simulink model "RL_controller_"  (R2022b)
settings: Solver=VariableStepAuto  StartTime=0.0  StopTime=inf  FixedStep=0.001  MaxStep=0.001  RelTol=1e-3
InitFcn:
  | ro = 0.1 ;
  | 
  | Ku = 9;
  | Tu = 4;
  | Kpmin = 0.32*Ku;
  | Kpmax = 0.6*Ku;
  | Kdmin = 0.08*Ku*Tu;
  | Kdmax = 0.15*Ku*Tu;
libraries: slpidlib x1, rllib x1, simulink x1
settings Model: SimulationMode=accelerator  Creator=Notebook  LastModifiedBy=Administrator
settings SolverCC: AlgebraicLoopSolver=TrustRegion
settings DebuggingCC: ArithmeticOperatorsInVariantConditions=warning
settings ModelReferenceCC: EnableRefExpFcnMdlSchedulingChecks=on
settings SFSimCC: CustomCodeUndefinedFunction=UseInterfaceOnly

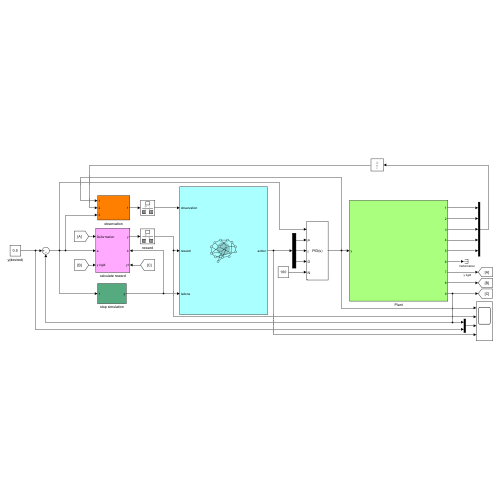
[thumbnail: Simulink's stored preview of the top-level diagram]
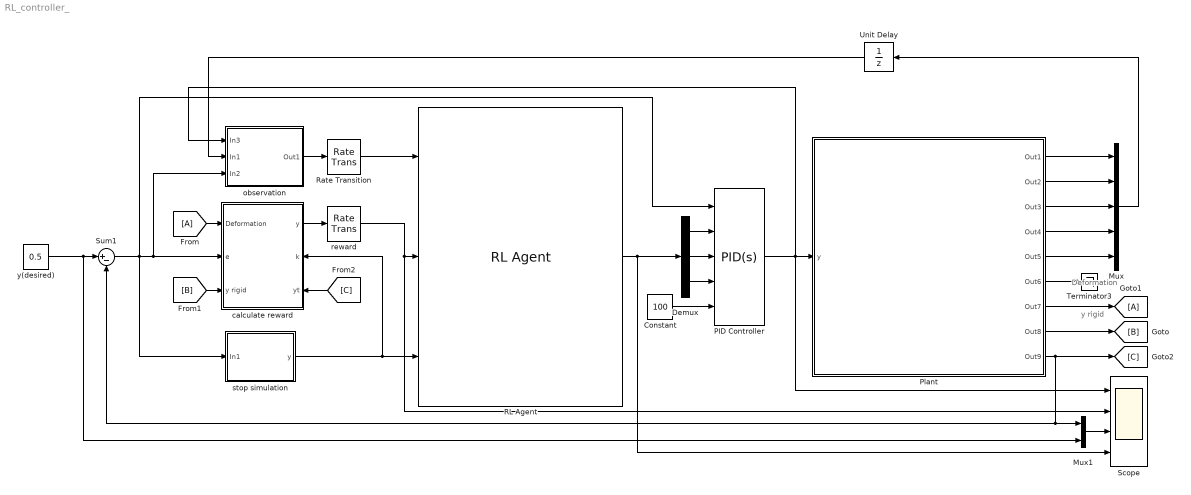
== system RL_controller_ ==
  note: Deformation
  note: y rigid
  Constant : Constant  Value=100
  Demux : Demux  Outputs=3
  From : From
  Goto1 : Goto
  Mux : Mux  Inputs=5
  Mux1 : Mux  Inputs=2
  PID Controller : slpidlib/PID Controller  Controller=PID  Form=Parallel  TimeDomain=Continuous-time  UseExternalTs=off  SampleTime=-1  IntegratorMethod=Forward Euler  FilterMethod=Forward Euler  ControllerParametersSource=external  P=1  I=1  UseKiTs=off  D=0  N=100  UseFilter=on  TunerSelectOption=Transfer Function Based (PID Tuner App)  InitialConditionSource=internal  InitialConditionForIntegrator=0  InitialConditionForFilter=0  DifferentiatorICPrevScaledInput=0  ExternalReset=none  TrackingMode=off  Kt=1  LimitOutput=off  SatLimitsSource=internal  UpperSaturationLimit=inf  LowerSaturationLimit=-inf  LinearizeAsGain=on  AntiWindupMode=none  Kb=1  LimitIntegrator=off  UpperIntegratorSaturationLimit=inf  LowerIntegratorSaturationLimit=-inf  POutMin=[]  POutMax=[]  IOutMin=[]  IOutMax=[]  DOutMin=[]  DOutMax=[]  NOutMin=[]  NOutMax=[]  SumOutMin=[]  SumOutMax=[]  SaturationOutMin=[]  SaturationOutMax=[]  PParamMin=[]  PParamMax=[]  IParamMin=[]  IParamMax=[]  DParamMin=[]  DParamMax=[]  NParamMin=[]  NParamMax=[]  KbParamMin=[]  KbParamMax=[]  KtParamMin=[]  KtParamMax=[]  KbOutMin=[]  KbOutMax=[]  KtOutMin=[]  KtOutMax=[]  IntegratorOutMin=[]  IntegratorOutMax=[]  FilterOutMin=[]  FilterOutMax=[]  SumI1OutMin=[]  SumI1OutMax=[]  SumI2OutMin=[]  SumI2OutMax=[]  SumI3OutMin=[]  SumI3OutMax=[]  SumI4OutMin=[]  SumI4OutMax=[]  SumDOutMin=[]  SumDOutMax=[]  DifferentiatorOutMin=[]  DifferentiatorOutMax=[]  FilterDiffOutCoefMin=[]  FilterDiffOutCoefMax=[]  ReciprocalOutMin=[]  ReciprocalOutMax=[]  SumDenOutMin=[]  SumDenOutMax=[]  SumNumOutMin=[]  SumNumOutMax=[]  DivideOutMin=[]  DivideOutMax=[]  UdiffTsProdOutMin=[]  UdiffTsProdOutMax=[]  NTsProdOutMin=[]  NTsProdOutMax=[]  UintegralTsProdOutMin=[]  UintegralTsProdOutMax=[]  UngainTsProdOutMin=[]  UngainTsProdOutMax=[]  ClampingZeroOutDataTypeStr=Inherit: Inherit via back propagation  ClampingZeroOutMin=[]  ClampingZeroOutMax=[]  FilterDenConstantOutDataTypeStr=Inherit: Inherit via back propagation  FilterDenConstantOutMin=[]  FilterDenConstantOutMax=[]  PCopyOutDataTypeStr=Inherit: Inherit via back propagation  PCopyOutMin=[]  PCopyOutMax=[]  NCopyOutDataTypeStr=Inherit: Inherit via back propagation  NCopyOutMin=[]  NCopyOutMax=[]  IntegratorContinuousStateAttributes=''  IntegratorStateMustResolveToSignalObject=off  IntegratorRTWStateStorageClass=Auto  FilterContinuousStateAttributes=''  FilterStateMustResolveToSignalObject=off  FilterRTWStateStorageClass=Auto  ParallelPVariant=ExternalParameters  IdealPVariant=Disabled  IVariant=ExternalParameters  DVariant=ExternalParameters  IntegratorVariant=Continuous  SatVariant=Disabled  AWVariant=Passthrough  PCopyVariant=Disabled  TRVariant=Disabled  FdbkBlocksVariant=Forward  IdealPFdbkVariant=Disabled  SatFdbkVariant=Disabled  DerivativeFilterVariant=ContFilter  NVariant=ExternalParameters  NCopyVariant=Disabled  FilterICVariant=InternalICsFilter  IntegratorICVariant=InternalICs  ExternalResetVariant=Disabled  TRSumVariant=Passthrough  SumFdbkVariant=Disabled  SumVariant=Sum_PID  TsampFilterVariant=InternalTs  TsampNgainVariant=Passthrough  TsampIntegralVariant=Passthrough  ExternalSaturationOutDataTypeStr=Inherit: Same as second input
  Plant : Subsystem
  RL Agent : rllib/RL Agent  Agent=agent  ExternalActionAsInput=off  ProvideLastAction=off  ProvideCumRwd=off  TreatAsDirectFeedthrough=on  UseStrictObservationDataTypes=off
  Rate Transition : RateTransition
  Scope : Scope  NumInputPorts=4
  Sum1 : Sum  Inputs=|+-
  Terminator3 : Terminator
  Unit Delay : UnitDelay  SampleTime=-1  HasFrameUpgradeWarning=on
  calculate reward : Subsystem
      settings: PortSchema="{\"entries\":[{\"content\":{\"sides\":[{\"content\":{\"connectorIds\":[\"In1\",\"In2\",\"In3\"]},\"type\":\"ConnectorPlacement.EquallySpacedRectSide\",\"uuid\":\"6d7fc479-8b54-4eda-9f6d-c70e7c76a1e2\"},{\"content\":{\"connectorIds\":[\"Out1\",\"In4\",\"In5\"],\"side\":\"RIGHT\"},\"type\":\"ConnectorPlacement.EquallySpacedRectSide\",\"uuid\":\"b691a02b-c792-4e07-977e-e9bf68ac6416\"},{\"content\":{\"connectorIds\":[],\"side\":\"TOP\"},\"type\":\"ConnectorPlacement.EquallySpacedRectSide\",\"uuid\":\"d0b1642a-ff91-438e-8bf3-0ab91db4c543\"}]},\"type\":\"ConnectorPlacement.EquallySpacedConnector\",\"uuid\":\"cdcc6e51-e785-4fe5-9481-e2f237055900\"}],\"packageUris\":[\"http://schema.mathworks.com/mf0/Connector/R2020b\"],\"version\":\"1.0\"}"
  observation : Subsystem
  reward : RateTransition
  stop simulation : Subsystem
  y(desired) : Constant  Value=0.5
  wires:
  Sum1/1 -> observation/3(In2), calculate reward/2(e), stop simulation/1(In1), PID Controller/1
  y(desired)/1 -> Mux1/2, Sum1/1
  calculate reward/1(y) -> reward/1
  observation/1(Out1) -> Rate Transition/1
  Rate Transition/1 -> RL Agent/1
  reward/1 -> RL Agent/2, Scope/2
  stop simulation/1(y) -> RL Agent/3, calculate reward/4(k)
  Plant/1(Out1) -> Mux/1
  Plant/2(Out2) -> Mux/2
  Plant/9(Out9) -> [C], Mux1/1, Sum1/2
  Plant/7(Out7) -> Goto1/1
  Plant/8(Out8) -> [B]
  From/1 -> calculate reward/1(Deformation)
  [B] -> calculate reward/3(y rigid)
  Mux/1 -> Unit Delay/1
  Mux1/1 -> Scope/3
  Plant/3(Out3) -> Mux/3
  [C] -> calculate reward/5(yt)
  Unit Delay/1 -> observation/2(In1)
  Plant/5(Out5) -> Mux/5
  Plant/6(Out6) -> Terminator3/1
  Plant/4(Out4) -> Mux/4
  PID Controller/1 -> observation/1(In3), Plant/1(y), Scope/1
  Demux/1 -> PID Controller/2
  Demux/2 -> PID Controller/3
  Demux/3 -> PID Controller/4
  RL Agent/1 -> Demux/1, Scope/4
  Constant/1 -> PID Controller/5

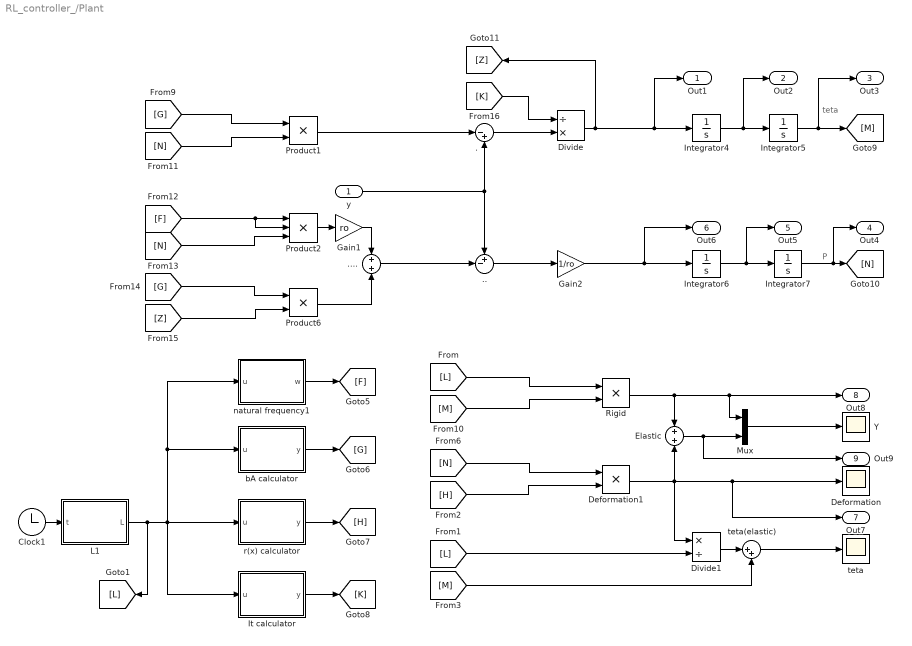
== system RL_controller_/Plant ==
  note: P
  note: teta
  y : Inport
  . : Sum  Inputs=|-+
  .. : Sum  Inputs=+-|
  .... : Sum  Inputs=+|+
  Clock1 : Clock
      settings: Decimation=2
  Deformation : Scope
  Deformation1 : Product
  Divide : Product  Inputs=/*
  Divide1 : Product  Inputs=*/
  Elastic : Sum  Inputs=+|+
  Gain1 : Gain  Gain=ro
  Gain2 : Gain  Gain=1/ro
  Integrator{4..7} (4 alike) : Integrator
  It calculator : MATLAB Function  TreatAsAtomicUnit=on
  L1 : MATLAB Function  TreatAsAtomicUnit=on
  Mux : Mux  Inputs=2
  Product1 : Product
  Product2 : Product  Inputs=3
  Product6 : Product
  Rigid : Product
  Y : Scope
  bA calculator : MATLAB Function  TreatAsAtomicUnit=on
  natural frequency1 : MATLAB Function  TreatAsAtomicUnit=on
  r(x) calculator : MATLAB Function  TreatAsAtomicUnit=on
  teta : Scope
  teta(elastic) : Sum  Inputs=|++
  Out1 : Outport
  Out2 : Outport  Port=2
  Out3 : Outport  Port=3
  Out4 : Outport  Port=4
  Out5 : Outport  Port=5
  Out6 : Outport  Port=6
  Out7 : Outport  Port=7
  Out8 : Outport  Port=8
  Out9 : Outport  Port=9
  wires:
  teta(elastic)/1 -> teta/1
  Integrator6/1 -> Out5/1, Integrator7/1
  [N] -> Product1/2
  [L] -> Rigid/1
  ./1 -> Divide/2
  [Z] -> Product6/2
  bA calculator/1(y) -> [G]
  Integrator7/1 -> Out4/1, [N]
  y/1 -> ./2, ../1
  ..../1 -> ../2
  Gain1/1 -> ..../1
  [G] -> Product1/1
  Product1/1 -> ./1
  [G] -> Product6/1
  [H] -> Deformation1/2
  Product2/1 -> Gain1/1
  [M] -> teta(elastic)/2
  [L] -> Divide1/2
  Rigid/1 -> Elastic/1, Out8/1, Mux/1
  Integrator4/1 -> Out2/1, Integrator5/1
  Divide1/1 -> teta(elastic)/1
  Mux/1 -> Y/1
  Elastic/1 -> Out9/1, Mux/2
  It calculator/1(y) -> [K]
  [N] -> Product2/3
  ../1 -> Gain2/1
  Integrator5/1 -> Out3/1, [M]
  natural frequency1/1(w) -> [F]
  Deformation1/1 -> Elastic/2, Out7/1, Deformation/1, Divide1/1
  [M] -> Rigid/2
  Clock1/1 -> L1/1(t)
  r(x) calculator/1(y) -> [H]
  [K] -> Divide/1
  [N] -> Deformation1/1
  L1/1(L) -> [L], r(x) calculator/1(u), It calculator/1(u), bA calculator/1(u), natural frequency1/1(u)
  Product6/1 -> ..../2
  Divide/1 -> [Z], Out1/1, Integrator4/1
  [F] -> Product2/1, Product2/2
  Gain2/1 -> Out6/1, Integrator6/1

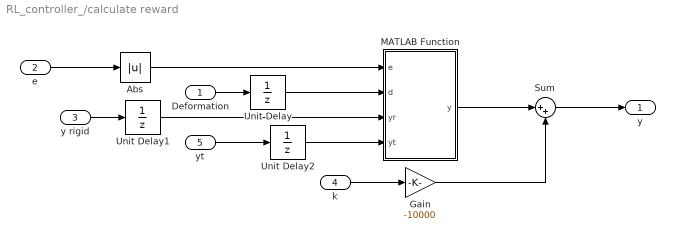
== system RL_controller_/calculate reward ==
  Deformation : Inport
  e : Inport  Port=2
  y rigid : Inport  Port=3
  k : Inport  Port=4
  yt : Inport  Port=5
  Abs : Abs  SaturateOnIntegerOverflow=off
  Gain : Gain  Gain=-10000
  MATLAB Function : MATLAB Function  TreatAsAtomicUnit=on
  Sum : Sum  Inputs=|++
  Unit Delay : UnitDelay  SampleTime=-1  HasFrameUpgradeWarning=on
  Unit Delay1 : UnitDelay  SampleTime=-1  HasFrameUpgradeWarning=on
  Unit Delay2 : UnitDelay  SampleTime=-1  HasFrameUpgradeWarning=on
  y : Outport
  wires:
  Deformation/1 -> Unit Delay/1
  y rigid/1 -> Unit Delay1/1
  Sum/1 -> y/1
  MATLAB Function/1(y) -> Sum/1
  Gain/1 -> Sum/2
  k/1 -> Gain/1
  Unit Delay/1 -> MATLAB Function/2(d)
  Unit Delay1/1 -> MATLAB Function/3(yr)
  yt/1 -> Unit Delay2/1
  Unit Delay2/1 -> MATLAB Function/4(yt)
  e/1 -> Abs/1
  Abs/1 -> MATLAB Function/1(e)

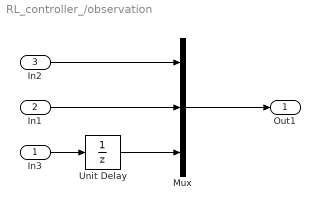
== system RL_controller_/observation ==
  In3 : Inport
  In1 : Inport  Port=2
  In2 : Inport  Port=3
  Mux : Mux  Inputs=3
  Unit Delay : UnitDelay  SampleTime=-1  HasFrameUpgradeWarning=on
  Out1 : Outport
  wires:
  Mux/1 -> Out1/1
  In1/1 -> Mux/2
  In2/1 -> Mux/1
  In3/1 -> Unit Delay/1
  Unit Delay/1 -> Mux/3

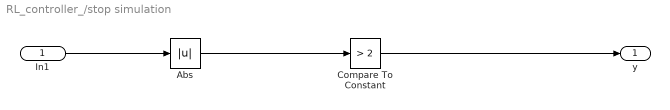
== system RL_controller_/stop simulation ==
  In1 : Inport
  Abs : Abs  SaturateOnIntegerOverflow=off
  Compare To Constant : simulink/Logic and Bit Operations/Compare To Constant  relop=>  const=2  OutDataTypeStr=boolean
  y : Outport
  wires:
  Abs/1 -> Compare To Constant/1
  In1/1 -> Abs/1
  Compare To Constant/1 -> y/1

== matlab function RL_controller_/calculate reward/MATLAB Function ==
  data: e input; y output; d input; yr input; yt input
function y = fcn(e,d,yr,yt)

w = 0 ; 
if e < 0.5 
    w = 1 ; 
end
if e < 0.05 
    w = 10 ; 
end


r = w - 5*(yr - 0.5)^2 - 5*abs(d) ;    

y = r;

== matlab function RL_controller_/Plant/It calculator ==
  data: u input; y output
function y = It_caculator(u) 

L = u ; 
Ih = 0.5 ; %kgm^2 
ro = 0.1 ; %kg/m 
It = Ih + (ro*L^3)/3 ; 


y = It  ;

== matlab function RL_controller_/Plant/L1 ==
  data: t input; L output
function L = fcn(t)

LL = 1 ; 
L = LL;

== matlab function RL_controller_/Plant/bA calculator ==
  data: u input; y output
function y = bA_caculator(u) 

L = u ; 
ro = 0.1 ; %kg/m 
a = (L)^(-0.5) ; 
A = 1.8751 ; 
b = (cosh(A)+cos(A))/(sinh(A)+sin(A)) ;  

x = 0:0.001:L ; 

bb = ro.*x.*a.*(cosh(A.*x./L) - cos(A.*x./L) + b*(sin(A.*x./L) - sinh(A.*x./L))) ;

bA = trapz(x,bb);

y = bA  ;

== matlab function RL_controller_/Plant/natural frequency1 ==
  data: u input; w output
function w = fcn(u)

L = u ; 
ro = 0.1 ; %kg/m 
EI = 2.0 ; %Nm^2 ; 
A = 1.8751 ; 

w = (A^2/L^2)*((EI)/(ro))^0.5 ;

== matlab function RL_controller_/Plant/r(x) calculator ==
  data: u input; y output
function y = r_caculator(u) 

L = u ; 
a = (L)^(-0.5) ; 
A = 1.8751 ; 
b = (cosh(A)+cos(A))/(sinh(A)+sin(A))  ; 

r = a*(cosh(A) - cos(A) + b*(sin(A) - sinh(A))) ;

y = r  ;
